simulink model "KeylessStart_harness"  (Simulink 7.7)
settings: Solver=FixedStepDiscrete  SolverMode=SingleTasking  StartTime=0.0  StopTime=100  FixedStep=.01  RelTol=1e-3
PostLoadFcn:
  | cd '..';
  | PostLoadFcn;
  | cd 'harness';
undefined symbols (not defined in the file): sigbuilder_block, srate
libraries: simulink x3
settings Model: Creator=smindema  LastModifiedBy=aliebel  CovMetricSettings=dcmw  CovHTMLOptions=-aTS=1 -bRG=1 -bTC=1 -hTR=0 -nFC=0 -scm=1 -bcm=1 -xEv=0  covSaveCumulativeToWorkspaceVar=off  CovSaveSingleToWorkspaceVar=off
settings MATStruct: SampleTime=0.01  Offset=0  Priority=[1.0]
settings DataIOCC: LimitDataPoints=off  SaveOutput=off  SaveTime=off
settings OptimizationCC: BlockReduction=off  InlineParams=on  ExpressionFolding=off  StateBitsets=on  DataBitsets=on  UseTempVars=on  InitFltsAndDblsToZero=on  NoFixptDivByZeroProtection=on  EfficientFloat2IntCast=on  OptimizeModelRefInitCode=on
settings DebuggingCC: SaveWithParameterizedLinksMsg=none  MultiTaskDSMMsg=warning  MultiTaskCondExecSysMsg=none  IntegerOverflowMsg=none  ModelReferenceCSMismatchMessage=warning
settings HardwareCC: ProdBitPerInt=16  ProdBitPerPointer=16  ProdIntDivRoundTo=Floor  ProdEndianess=BigEndian  ProdWordSize=16  ProdHWDeviceType=Motorola HC12
settings ModelReferenceCC: ModelReferenceNumInstancesAllowed=Single
settings RTWCC: SystemTargetFile=ert.tlc  GenCodeOnly=on  TemplateMakefile=ert_default_tmf  Description=Real-Time Workshop Embedded Coder (no auto configuration)  GenerateReport=on  RetainRTWFile=on  ProcessScript=ert_make_rtw_hook  IncludeHyperlinkInReport=on  LaunchReport=on  IncludeERTFirstTime=on
settings RTWCC: CustomHeaderCode=|
  | #include "cpp_req_defines.h"
  | #include "hw_fin.h"
  | #include "cdata.h"
settings CodeAppCC: IgnoreCustomStorageClasses=off  DefineNamingRule=UpperCase
settings ERTTargetCC: TargetFcnLib=ansi_tfl_tmw.mat  FunctionExecutionProfile=off  MultiwordLength=2048  GenerateSampleERTMain=on  IncludeMdlTerminateFcn=off  SupportAbsoluteTime=off  SupportNonFinite=off  SupportComplex=off  PurelyIntegerCode=on  ERTCustomFileTemplate=gen_rtw_req_defines_h.tlc  GlobalDataDefinition=InSeparateSourceFile  GlobalDataReference=InSeparateHeaderFile  ConvertIfToSwitch=off

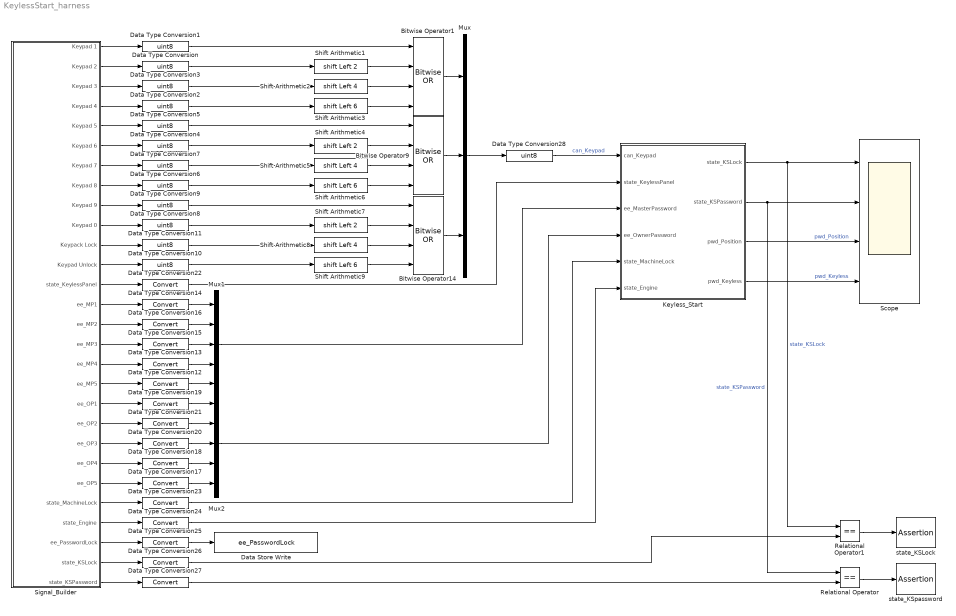
== system KeylessStart_harness ==
  Bitwise Operator1 : simulink/Logic and Bit Operations/Bitwise Operator  logicop=OR  UseBitMask=off  NumInputPorts=4  BitMask=bin2dec('11011001')  BitMaskRealWorld=Stored Integer
  Bitwise Operator14 : simulink/Logic and Bit Operations/Bitwise Operator  logicop=OR  UseBitMask=off  NumInputPorts=4  BitMask=bin2dec('11011001')  BitMaskRealWorld=Stored Integer
  Bitwise Operator9 : simulink/Logic and Bit Operations/Bitwise Operator  logicop=OR  UseBitMask=off  NumInputPorts=4  BitMask=bin2dec('11011001')  BitMaskRealWorld=Stored Integer
  Data Store Write : DataStoreWrite  DataStoreName=ee_PasswordLock
  Data Type Conversion{,1..11,28} (13 alike) : DataTypeConversion  OutDataTypeStr=uint8
  Data Type Conversion{12..27} (16 alike) : DataTypeConversion
  Keyless_Start : Subsystem  TreatAsAtomicUnit=on  SystemSampleTime=srate  RTWFileName=mod_System
      settings: RTWSystemCode=Function  RTWFileNameOpts=User specified
  Mux : Mux  Inputs=3
  Mux1 : Mux  Inputs=5
  Mux2 : Mux  Inputs=5
  Relational Operator : RelationalOperator  Operator===  OutDataTypeStr=boolean
  Relational Operator1 : RelationalOperator  Operator===  OutDataTypeStr=boolean
  Scope : Scope  NumInputPorts=4
      settings: TimeRange=100  YMin=0~0~0~0  YMax=6~10~6~60  DataFormat=Array
  Shift Arithmetic1 : ArithShift  BitShiftNumber=2  BitShiftDirection=Left
  Shift Arithmetic2 : ArithShift  BitShiftNumber=4  BitShiftDirection=Left
  Shift Arithmetic3 : ArithShift  BitShiftNumber=6  BitShiftDirection=Left
  Shift Arithmetic4 : ArithShift  BitShiftNumber=2  BitShiftDirection=Left
  Shift Arithmetic5 : ArithShift  BitShiftNumber=4  BitShiftDirection=Left
  Shift Arithmetic6 : ArithShift  BitShiftNumber=6  BitShiftDirection=Left
  Shift Arithmetic7 : ArithShift  BitShiftNumber=2  BitShiftDirection=Left
  Shift Arithmetic8 : ArithShift  BitShiftNumber=4  BitShiftDirection=Left
  Shift Arithmetic9 : ArithShift  BitShiftNumber=6  BitShiftDirection=Left
  Signal_Builder : Subsystem  Tag=STV Subsys  LoadFcn=sigbuilder_block('load');  StartFcn=sigbuilder_block('start');  StopFcn=sigbuilder_block('stop');  ClipboardFcn=sigbuilder_block('clipboard');  mask(Sigbuilder block){}
      mask help: Sigbuilder GUI
      mask init:
      | if ~strcmp(get_param(bdroot(gcbh),'SimulationStatus'),'stopped') tuvar = sigbuilder_block('maskInit'); end
      settings: CopyFcn=sigbuilder_block('copy');  DeleteFcn=sigbuilder_block('delete');  ModelCloseFcn=sigbuilder_block('modelClose');  PreSaveFcn=sigbuilder_block('preSave');  NameChangeFcn=sigbuilder_block('namechange');  OpenFcn=sigbuilder_block('open',[126.75 84.75 1007.25 697.5 ]);  CloseFcn=sigbuilder_block('close');
      mask Display: plot(0,0,100,100,[10,10,40,40,10],[80,20,20,80,80],[40,10],[50,50], [40,27,10],[65,72,56],[40,25,25,10],[28,28,43,43]);
  state_KSLock : Assertion  Enabled=off
  state_KSpassword : Assertion  Enabled=off
  wires:
  Signal_Builder/2(Keypad 2) -> Data Type Conversion/1
  Relational Operator/1 -> state_KSpassword/1
  Signal_Builder/1(Keypad 1) -> Data Type Conversion1/1
  Bitwise Operator1/1 -> Mux/1
  Shift Arithmetic1/1 -> Bitwise Operator1/2
  Shift Arithmetic2/1 -> Bitwise Operator1/3
  Shift Arithmetic3/1 -> Bitwise Operator1/4
  Shift Arithmetic4/1 -> Bitwise Operator9/2
  Shift Arithmetic5/1 -> Bitwise Operator9/3
  Shift Arithmetic6/1 -> Bitwise Operator9/4
  Bitwise Operator9/1 -> Mux/2
  Bitwise Operator14/1 -> Mux/3
  Shift Arithmetic7/1 -> Bitwise Operator14/2
  Shift Arithmetic8/1 -> Bitwise Operator14/3
  Shift Arithmetic9/1 -> Bitwise Operator14/4
  Mux/1 -> Data Type Conversion28/1
  Data Type Conversion1/1 -> Bitwise Operator1/1
  Signal_Builder/4(Keypad 4) -> Data Type Conversion2/1
  Signal_Builder/5(Keypad 5) -> Data Type Conversion5/1
  Signal_Builder/6(Keypad 6) -> Data Type Conversion4/1
  Signal_Builder/7(Keypad 7) -> Data Type Conversion7/1
  Signal_Builder/8(Keypad 8) -> Data Type Conversion6/1
  Signal_Builder/9(Keypad 9) -> Data Type Conversion9/1
  Signal_Builder/11(Keypack Lock) -> Data Type Conversion11/1
  Signal_Builder/12(Keypad Unlock) -> Data Type Conversion10/1
  Signal_Builder/13(state_KeylessPanel) -> Data Type Conversion22/1
  Mux1/1 -> Keyless_Start/3(ee_MasterPassword)
  Signal_Builder/14(ee_MP1) -> Data Type Conversion14/1
  Signal_Builder/15(ee_MP2) -> Data Type Conversion16/1
  Signal_Builder/16(ee_MP3) -> Data Type Conversion15/1
  Signal_Builder/17(ee_MP4) -> Data Type Conversion13/1
  Signal_Builder/18(ee_MP5) -> Data Type Conversion12/1
  Data Type Conversion14/1 -> Mux1/1
  Data Type Conversion16/1 -> Mux1/2
  Data Type Conversion15/1 -> Mux1/3
  Data Type Conversion13/1 -> Mux1/4
  Data Type Conversion12/1 -> Mux1/5
  Data Type Conversion19/1 -> Mux2/1
  Data Type Conversion21/1 -> Mux2/2
  Data Type Conversion20/1 -> Mux2/3
  Data Type Conversion18/1 -> Mux2/4
  Data Type Conversion17/1 -> Mux2/5
  Signal_Builder/19(ee_OP1) -> Data Type Conversion19/1
  Signal_Builder/20(ee_OP2) -> Data Type Conversion21/1
  Signal_Builder/21(ee_OP3) -> Data Type Conversion20/1
  Signal_Builder/22(ee_OP4) -> Data Type Conversion18/1
  Signal_Builder/23(ee_OP5) -> Data Type Conversion17/1
  Mux2/1 -> Keyless_Start/4(ee_OwnerPassword)
  Signal_Builder/24(state_MachineLock) -> Data Type Conversion23/1
  Signal_Builder/25(state_Engine) -> Data Type Conversion24/1
  Keyless_Start/1(state_KSLock) -> Scope/1, Relational Operator1/1  "state_KSLock"
  Keyless_Start/2(state_KSPassword) -> Relational Operator/1, Scope/2  "state_KSPassword"
  Keyless_Start/3(pwd_Position) -> Scope/3  "pwd_Position"
  Keyless_Start/4(pwd_Keyless) -> Scope/4  "pwd_Keyless"
  Signal_Builder/26(ee_PasswordLock) -> Data Type Conversion25/1
  Relational Operator1/1 -> state_KSLock/1
  Signal_Builder/27(state_KSLock) -> Data Type Conversion26/1
  Signal_Builder/28(state_KSPassword) -> Data Type Conversion27/1
  Data Type Conversion22/1 -> Keyless_Start/2(state_KeylessPanel)
  Data Type Conversion23/1 -> Keyless_Start/5(state_MachineLock)
  Data Type Conversion24/1 -> Keyless_Start/6(state_Engine)
  Data Type Conversion25/1 -> Data Store Write/1
  Data Type Conversion26/1 -> Relational Operator1/2
  Data Type Conversion27/1 -> Relational Operator/2
  Data Type Conversion28/1 -> Keyless_Start/1(can_Keypad)  "can_Keypad"
  Data Type Conversion/1 -> Shift Arithmetic1/1
  Data Type Conversion3/1 -> Shift Arithmetic2/1
  Data Type Conversion2/1 -> Shift Arithmetic3/1
  Data Type Conversion4/1 -> Shift Arithmetic4/1
  Data Type Conversion7/1 -> Shift Arithmetic5/1
  Data Type Conversion6/1 -> Shift Arithmetic6/1
  Data Type Conversion8/1 -> Shift Arithmetic7/1
  Data Type Conversion11/1 -> Shift Arithmetic8/1
  Data Type Conversion10/1 -> Shift Arithmetic9/1
  Data Type Conversion9/1 -> Bitwise Operator14/1
  Data Type Conversion5/1 -> Bitwise Operator9/1
  Signal_Builder/10(Keypad 0) -> Data Type Conversion8/1
  Signal_Builder/3(Keypad 3) -> Data Type Conversion3/1

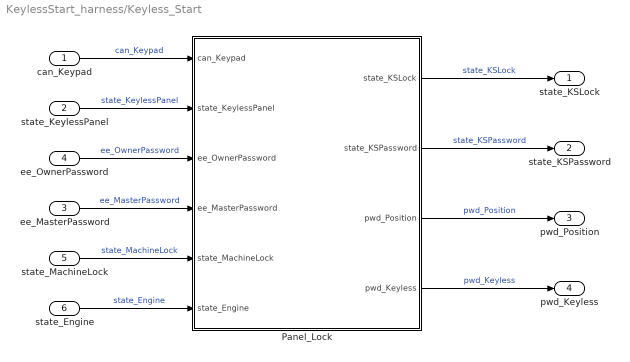
== system KeylessStart_harness/Keyless_Start ==
  can_Keypad : Inport
  state_KeylessPanel : Inport  Port=2
  ee_MasterPassword : Inport  Port=3
  ee_OwnerPassword : Inport  Port=4
  state_MachineLock : Inport  Port=5
  state_Engine : Inport  Port=6
  Panel_Lock : Stateflow chart  TreatAsAtomicUnit=on
  state_KSLock : Outport
  state_KSPassword : Outport  Port=2
  pwd_Position : Outport  Port=3
  pwd_Keyless : Outport  Port=4
  wires:
  can_Keypad/1 -> Panel_Lock/1(can_Keypad)  "can_Keypad"
  state_KeylessPanel/1 -> Panel_Lock/2(state_KeylessPanel)  "state_KeylessPanel"
  Panel_Lock/1(state_KSLock) -> state_KSLock/1  "state_KSLock"
  state_MachineLock/1 -> Panel_Lock/5(state_MachineLock)  "state_MachineLock"
  Panel_Lock/2(state_KSPassword) -> state_KSPassword/1  "state_KSPassword"
  Panel_Lock/3(pwd_Position) -> pwd_Position/1  "pwd_Position"
  Panel_Lock/4(pwd_Keyless) -> pwd_Keyless/1  "pwd_Keyless"
  state_Engine/1 -> Panel_Lock/6(state_Engine)  "state_Engine"
  ee_OwnerPassword/1 -> Panel_Lock/3(ee_OwnerPassword)  "ee_OwnerPassword"
  ee_MasterPassword/1 -> Panel_Lock/4(ee_MasterPassword)  "ee_MasterPassword"

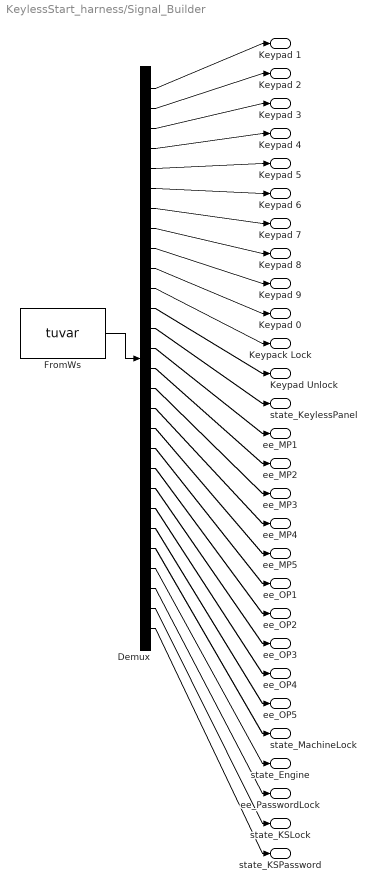
== system KeylessStart_harness/Signal_Builder ==
  Demux : Demux  Tag=STV Demux  Outputs=28
  FromWs : FromWorkspace  Tag=STV FromWs  VariableName=tuvar  SampleTime=0  SigBuilderData=DataTag0  VnvData=DataTag1
      SigBuilderData=|
      | common.afterFinalStr = 'Extrapolate'
      | common.sampleTime = 0
      | dataSet(1).timeRange = [0 100]
      | dataSet(1).name = 'Keypad'
      | dataSet(2).timeRange = [0 100]
      | dataSet(2).name = 'Password'
      | dataSet(3).timeRange = [0 100]
      | dataSet(3).name = 'Password1'
      | dataSet(4).timeRange = [0 100]
      | dataSet(4).name = 'Password2'
      | dataSet(5).timeRange = [0 100]
      | dataSet(5).name = 'Lock'
      | sbobj.Groups(1).Name = 'Keypad'
      | sbobj.Groups(1).Signals(1).Name = 'Keypad 1'
      | sbobj.Groups(1).Signals(1).XData = [0 25 25 26 26 100]
      | sbobj.Groups(1).Signals(1).YData = [0 0 1 1 0 0]
      | sbobj.Groups(1).Signals(2).Name = 'Keypad 2'
      | sbobj.Groups(1).Signals(2).XData = [0 23 23 24 24 100]
      | sbobj.Groups(1).Signals(2).YData = [0 0 1 1 0 0]
      | sbobj.Groups(1).Signals(3).Name = 'Keypad 3'
      | sbobj.Groups(1).Signals(3).XData = [0 21 21 22 22 100]
      | sbobj.Groups(1).Signals(3).YData = [0 0 1 1 0 0]
      | sbobj.Groups(1).Signals(4).Name = 'Keypad 4'
      | sbobj.Groups(1).Signals(4).XData = [0 19 19 20 20 100]
      | sbobj.Groups(1).Signals(4).YData = [0 0 1 1 0 0]
      | sbobj.Groups(1).Signals(5).Name = 'Keypad 5'
      | sbobj.Groups(1).Signals(5).XData = [0 17 17 18 18 100]
      | sbobj.Groups(1).Signals(5).YData = [0 0 1 1 0 0]
      | sbobj.Groups(1).Signals(6).Name = 'Keypad 6'
      | sbobj.Groups(1).Signals(6).XData = [0 13 13 14 14 100]
      | sbobj.Groups(1).Signals(6).YData = [0 0 1 1 0 0]
      | sbobj.Groups(1).Signals(7).Name = 'Keypad 7'
      | sbobj.Groups(1).Signals(7).XData = [0 11 11 12 12 100]
      | sbobj.Groups(1).Signals(7).YData = [0 0 1 1 0 0]
      | sbobj.Groups(1).Signals(8).Name = 'Keypad 8'
      | sbobj.Groups(1).Signals(8).XData = [0 9 9 10 10 100]
      | sbobj.Groups(1).Signals(8).YData = [0 0 1 1 0 0]
      | sbobj.Groups(1).Signals(9).Name = 'Keypad 9'
      | sbobj.Groups(1).Signals(9).XData = [0 7 7 8 8 50 50 51 51 52 52 53 53 54 54 55 55 56 56 57 57 58 58 59 59 61 61 62 62 63 63 64 64 65 65 66 66 67 67 68 68 69 69 70 70 100]
      | sbobj.Groups(1).Signals(9).YData = [0 0 1 1 0 0 1 1 0 0 1 1 0 0 1 1 0 0 1 1 0 0 1 1 0 0 1 1 0 0 1 1 0 0 1 1 0 0 1 1 0 0 1 1 0 0]
      | sbobj.Groups(1).Signals(10).Name = 'Keypad 0'
      | sbobj.Groups(1).Signals(10).XData = [0 5 5 6 6 29 29 30 30 31 31 32 32 33 33 34 34 35 35 36 36 37 37 38 38 100]
      | sbobj.Groups(1).Signals(10).YData = [0 0 1 1 0 0 1 1 0 0 1 1 0 0 1 1 0 0 1 1 0 0 1 1 0 0]
      | sbobj.Groups(1).Signals(11).Name = 'Keypack Lock'
      | sbobj.Groups(1).Signals(11).XData = [0 2 2 4 4 15 15 16 16 27 27 28 28 40 40 41 41 42 42 46 46 100]
      | sbobj.Groups(1).Signals(11).YData = [0 0 1 1 0 0 1 1 0 0 1 1 0 0 1 1 0 0 1 1 0 0]
      | sbobj.Groups(1).Signals(12).Name = 'Keypad Unlock'
      | sbobj.Groups(1).Signals(12).XData = [0 2 2 3 3 40 40 41 41 43 43 46 46 100]
      | sbobj.Groups(1).Signals(12).YData = [0 0 1 1 0 0 1 1 0 0 1 1 0 0]
      | sbobj.Groups(1).Signals(13).Name = 'state_KeylessPanel'
      | sbobj.Groups(1).Signals(13).XData = [0 100]
      | sbobj.Groups(1).Signals(13).YData = [8 8]
      | sbobj.Groups(1).Signals(14).Name = 'ee_MP1'
      | sbobj.Groups(1).Signals(14).XData = [0 100]
      | sbobj.Groups(1).Signals(14).YData = [48 48]
      | sbobj.Groups(1).Signals(15).Name = 'ee_MP2'
      | sbobj.Groups(1).Signals(15).XData = [0 100]
      | sbobj.Groups(1).Signals(15).YData = [48 48]
      | sbobj.Groups(1).Signals(16).Name = 'ee_MP3'
      | sbobj.Groups(1).Signals(16).XData = [0 100]
      | sbobj.Groups(1).Signals(16).YData = [48 48]
      | sbobj.Groups(1).Signals(17).Name = 'ee_MP4'
      | sbobj.Groups(1).Signals(17).XData = [0 100]
      | sbobj.Groups(1).Signals(17).YData = [48 48]
      | sbobj.Groups(1).Signals(18).Name = 'ee_MP5'
      | sbobj.Groups(1).Signals(18).XData = [0 100]
      | sbobj.Groups(1).Signals(18).YData = [48 48]
      | sbobj.Groups(1).Signals(19).Name = 'ee_OP1'
      | sbobj.Groups(1).Signals(19).XData = [0 100]
      | sbobj.Groups(1).Signals(19).YData = [0 0]
      | sbobj.Groups(1).Signals(20).Name = 'ee_OP2'
      | sbobj.Groups(1).Signals(20).XData = [0 100]
      | sbobj.Groups(1).Signals(20).YData = [0 0]
      | sbobj.Groups(1).Signals(21).Name = 'ee_OP3'
      | sbobj.Groups(1).Signals(21).XData = [0 100]
      | sbobj.Groups(1).Signals(21).YData = [0 0]
      | sbobj.Groups(1).Signals(22).Name = 'ee_OP4'
      | sbobj.Groups(1).Signals(22).XData = [0 100]
      | sbobj.Groups(1).Signals(22).YData = [0 0]
      | sbobj.Groups(1).Signals(23).Name = 'ee_OP5'
      | sbobj.Groups(1).Signals(23).XData = [0 100]
      | sbobj.Groups(1).Signals(23).YData = [0 0]
      | sbobj.Groups(1).Signals(24).Name = 'state_MachineLock'
      | sbobj.Groups(1).Signals(24).XData = [0 37.02 37.02 37.03 37.03 100]
      | sbobj.Groups(1).Signals(24).YData = [0 0 1 1 0 0]
      | sbobj.Groups(1).Signals(25).Name = 'state_Engine'
      | sbobj.Groups(1).Signals(25).XData = [0 1 1 100]
      | sbobj.Groups(1).Signals(25).YData = [0 0 1 1]
      | sbobj.Groups(1).Signals(26).Name = 'ee_PasswordLock'
      | sbobj.Groups(1).Signals(26).XData = [0 37.02 37.02 100]
      | sbobj.Groups(1).Signals(26).YData = [0 0 1 1]
      | sbobj.Groups(1).Signals(27).Name = 'state_KSLock'
      | sbobj.Groups(1).Signals(27).XData = [0 0.01 0.02 0.03 0.04 0.05 0.06 0.07 0.08 0.09 0.1 0.11 ... (10001 elements, 1x10001)]
      | sbobj.Groups(1).Signals(27).YData = [0 0 0 0 0 0 0 0 0 0 0 0 ... (10001 elements, 1x10001)]
      | sbobj.Groups(1).Signals(28).Name = 'state_KSPassword'
      | sbobj.Groups(1).Signals(28).XData = [0 0.01 0.02 0.03 0.04 0.05 0.06 0.07 0.08 0.09 0.1 0.11 ... (10001 elements, 1x10001)]
      | sbobj.Groups(1).Signals(28).YData = [0 0 0 0 0 0 0 0 0 0 0 0 ... (10001 elements, 1x10001)]
      | sbobj.Groups(1).TimeRange = [0 100]
      | sbobj.Groups(2).Name = 'Password'
      | sbobj.Groups(2).Signals(1).Name = 'Keypad 1'
      | sbobj.Groups(2).Signals(1).XData = [0 37 37 38 38 49 49 50 50 61 61 62 62 85 85 86 86 100]
      | sbobj.Groups(2).Signals(1).YData = [0 0 1 1 0 0 1 1 0 0 1 1 0 0 1 1 0 0]
      | sbobj.Groups(2).Signals(2).Name = 'Keypad 2'
      | sbobj.Groups(2).Signals(2).XData = [0 51 51 52 52 63 63 64 64 87 87 88 88 100]
      | sbobj.Groups(2).Signals(2).YData = [0 0 1 1 0 0 1 1 0 0 1 1 0 0]
      | sbobj.Groups(2).Signals(3).Name = 'Keypad 3'
      | sbobj.Groups(2).Signals(3).XData = [0 55 55 56 56 65 65 66 66 89 89 90 90 100]
      | sbobj.Groups(2).Signals(3).YData = [0 0 1 1 0 0 1 1 0 0 1 1 0 0]
      | sbobj.Groups(2).Signals(4).Name = 'Keypad 4'
      | sbobj.Groups(2).Signals(4).XData = [0 53 53 54 54 69 69 70 70 91 91 92 92 100]
      | sbobj.Groups(2).Signals(4).YData = [0 0 1 1 0 0 1 1 0 0 1 1 0 0]
      | sbobj.Groups(2).Signals(5).Name = 'Keypad 5'
      | sbobj.Groups(2).Signals(5).XData = [0 57 57 58 58 67 67 68 68 93 94 100]
      | sbobj.Groups(2).Signals(5).YData = [0 0 1 1 0 0 1 1 0 0 0 0]
      | sbobj.Groups(2).Signals(6).Name = 'Keypad 6'
      | sbobj.Groups(2).Signals(6).XData = [0 39 39 40 40 100]
      | sbobj.Groups(2).Signals(6).YData = [0 0 1 1 0 0]
      | sbobj.Groups(2).Signals(7).Name = 'Keypad 7'
      | sbobj.Groups(2).Signals(7).XData = [0 41 41 42 42 100]
      | sbobj.Groups(2).Signals(7).YData = [0 0 1 1 0 0]
      | sbobj.Groups(2).Signals(8).Name = 'Keypad 8'
      | sbobj.Groups(2).Signals(8).XData = [0 43 43 44 44 100]
      | sbobj.Groups(2).Signals(8).YData = [0 0 1 1 0 0]
      | sbobj.Groups(2).Signals(9).Name = 'Keypad 9'
      | sbobj.Groups(2).Signals(9).XData = [0 30 30 33 33 45 45 46 46 77 77 78 78 79 79 80 80 81 81 82 82 100]
      | sbobj.Groups(2).Signals(9).YData = [0 0 1 1 0 0 1 1 0 0 1 1 0 0 1 1 0 0 1 1 0 0]
      | sbobj.Groups(2).Signals(10).Name = 'Keypad 0'
      | sbobj.Groups(2).Signals(10).XData = [0 3 3 4 4 22 22 23 23 24 24 25 25 26 26 27 27 28 28 29 29 30 33 73 73 74 74 75 75 76 76 93 93 94 94 100]
      | sbobj.Groups(2).Signals(10).YData = [0 0 1 1 0 0 1 1 0 0 1 1 0 0 1 1 0 0 1 1 0 0 0 0 1 1 0 0 1 1 0 0 1 1 0 0]
      | sbobj.Groups(2).Signals(11).Name = 'Keypack Lock'
      | sbobj.Groups(2).Signals(11).XData = [0 1 1 2 2 20 20 21 21 35 35 36 36 47 47 48 48 59 59 60 60 71 71 72 72 83 83 84 84 100]
      | sbobj.Groups(2).Signals(11).YData = [0 0 1 1 0 0 1 1 0 0 1 1 0 0 1 1 0 0 1 1 0 0 1 1 0 0 1 1 0 0]
      | sbobj.Groups(2).Signals(12).Name = 'Keypad Unlock'
      | sbobj.Groups(2).Signals(12).XData = [0 100]
      | sbobj.Groups(2).Signals(12).YData = [0 0]
      | sbobj.Groups(2).Signals(13).Name = 'state_KeylessPanel'
      | sbobj.Groups(2).Signals(13).XData = [0 100]
      | sbobj.Groups(2).Signals(13).YData = [8 8]
      | sbobj.Groups(2).Signals(14).Name = 'ee_MP1'
      | sbobj.Groups(2).Signals(14).XData = [0 100]
      | sbobj.Groups(2).Signals(14).YData = [48 48]
      | sbobj.Groups(2).Signals(15).Name = 'ee_MP2'
      | sbobj.Groups(2).Signals(15).XData = [0 100]
      | sbobj.Groups(2).Signals(15).YData = [48 48]
      | sbobj.Groups(2).Signals(16).Name = 'ee_MP3'
      | sbobj.Groups(2).Signals(16).XData = [0 100]
      | sbobj.Groups(2).Signals(16).YData = [48 48]
      | sbobj.Groups(2).Signals(17).Name = 'ee_MP4'
      | sbobj.Groups(2).Signals(17).XData = [0 100]
      | sbobj.Groups(2).Signals(17).YData = [48 48]
      | sbobj.Groups(2).Signals(18).Name = 'ee_MP5'
      | sbobj.Groups(2).Signals(18).XData = [0 100]
      | sbobj.Groups(2).Signals(18).YData = [48 48]
      | sbobj.Groups(2).Signals(19).Name = 'ee_OP1'
      | sbobj.Groups(2).Signals(19).XData = [0 100]
      | sbobj.Groups(2).Signals(19).YData = [49 49]
      | sbobj.Groups(2).Signals(20).Name = 'ee_OP2'
      | sbobj.Groups(2).Signals(20).XData = [0 100]
      | sbobj.Groups(2).Signals(20).YData = [50 50]
      | sbobj.Groups(2).Signals(21).Name = 'ee_OP3'
      | sbobj.Groups(2).Signals(21).XData = [0 100]
      | sbobj.Groups(2).Signals(21).YData = [51 51]
      | sbobj.Groups(2).Signals(22).Name = 'ee_OP4'
      | sbobj.Groups(2).Signals(22).XData = [0 100]
      | sbobj.Groups(2).Signals(22).YData = [52 52]
      | sbobj.Groups(2).Signals(23).Name = 'ee_OP5'
      | sbobj.Groups(2).Signals(23).XData = [0 100]
      | sbobj.Groups(2).Signals(23).YData = [53 53]
      | sbobj.Groups(2).Signals(24).Name = 'state_MachineLock'
      | sbobj.Groups(2).Signals(24).XData = [0 100]
      | sbobj.Groups(2).Signals(24).YData = [0 0]
      | sbobj.Groups(2).Signals(25).Name = 'state_Engine'
      | sbobj.Groups(2).Signals(25).XData = [0 1 1 100]
      | sbobj.Groups(2).Signals(25).YData = [0 0 1 1]
      | sbobj.Groups(2).Signals(26).Name = 'ee_PasswordLock'
      | sbobj.Groups(2).Signals(26).XData = [0 100]
      | sbobj.Groups(2).Signals(26).YData = [0 0]
      | sbobj.Groups(2).Signals(27).Name = 'state_KSLock'
      | sbobj.Groups(2).Signals(27).XData = [0 0.01 0.02 0.03 0.04 0.05 0.06 0.07 0.08 0.09 0.1 0.11 ... (10001 elements, 1x10001)]
      | sbobj.Groups(2).Signals(27).YData = [0 0 0 0 0 0 0 0 0 0 0 0 ... (10001 elements, 1x10001)]
      | sbobj.Groups(2).Signals(28).Name = 'state_KSPassword'
      | sbobj.Groups(2).Signals(28).XData = [0 0.01 0.02 0.03 0.04 0.05 0.06 0.07 0.08 0.09 0.1 0.11 ... (10001 elements, 1x10001)]
      | sbobj.Groups(2).Signals(28).YData = [0 0 0 0 0 0 0 0 0 0 0 0 ... (10001 elements, 1x10001)]
      | sbobj.Groups(2).TimeRange = [0 100]
      | sbobj.Groups(3).Name = 'Password1'
      | sbobj.Groups(3).Signals(1).Name = 'Keypad 1'
      | sbobj.Groups(3).Signals(1).XData = [0 15 15 16 16 49 50 61 62 85 86 100]
      | sbobj.Groups(3).Signals(1).YData = [0 0 1 1 0 0 0 0 0 0 0 0]
      | sbobj.Groups(3).Signals(2).Name = 'Keypad 2'
      | sbobj.Groups(3).Signals(2).XData = [0 17 17 18 18 63 64 87 88 100]
      | sbobj.Groups(3).Signals(2).YData = [0 0 1 1 0 0 0 0 0 0]
      | sbobj.Groups(3).Signals(3).Name = 'Keypad 3'
      | sbobj.Groups(3).Signals(3).XData = [0 19 19 20 20 65 66 89 90 100]
      | sbobj.Groups(3).Signals(3).YData = [0 0 1 1 0 0 0 0 0 0]
      | sbobj.Groups(3).Signals(4).Name = 'Keypad 4'
      | sbobj.Groups(3).Signals(4).XData = [0 21 21 22 22 69 70 91 92 100]
      | sbobj.Groups(3).Signals(4).YData = [0 0 1 1 0 0 0 0 0 0]
      | sbobj.Groups(3).Signals(5).Name = 'Keypad 5'
      | sbobj.Groups(3).Signals(5).XData = [0 23 23 24 24 67 68 93 94 100]
      | sbobj.Groups(3).Signals(5).YData = [0 0 1 1 0 0 0 0 0 0]
      | sbobj.Groups(3).Signals(6).Name = 'Keypad 6'
      | sbobj.Groups(3).Signals(6).XData = [0 39 40 100]
      | sbobj.Groups(3).Signals(6).YData = [0 0 0 0]
      | sbobj.Groups(3).Signals(7).Name = 'Keypad 7'
      | sbobj.Groups(3).Signals(7).XData = [0 41 42 100]
      | sbobj.Groups(3).Signals(7).YData = [0 0 0 0]
      | sbobj.Groups(3).Signals(8).Name = 'Keypad 8'
      | sbobj.Groups(3).Signals(8).XData = [0 43 44 100]
      | sbobj.Groups(3).Signals(8).YData = [0 0 0 0]
      | sbobj.Groups(3).Signals(9).Name = 'Keypad 9'
      | sbobj.Groups(3).Signals(9).XData = [0 9 9 10 10 11 11 12 12 63 63 64 64 79 80 97 97 98 98 100]
      | sbobj.Groups(3).Signals(9).YData = [0 0 1 1 0 0 1 1 0 0 1 1 0 0 0 0 1 1 0 0]
      | sbobj.Groups(3).Signals(10).Name = 'Keypad 0'
      | sbobj.Groups(3).Signals(10).XData = [0 3 3 4 4 5 5 6 6 7 7 8 8 47 47 48 48 49 49 50 50 51 51 52 52 53 53 54 54 55 55 56 56 61 61 62 62 65 65 66 66 67 67 68 68 69 69 70 70 75 76 77 78 81 82 83 84 89 89 90 90 91 91 92 92 93 93 94 94 95 95 96 96 100]
      | sbobj.Groups(3).Signals(10).YData = [0 0 1 1 0 0 1 1 0 0 1 1 0 0 1 1 0 0 1 1 0 0 1 1 0 0 1 1 0 0 1 1 0 0 1 1 0 0 1 1 0 0 1 1 0 0 1 1 0 0 0 0 0 0 0 0 0 0 1 1 0 0 1 1 0 0 1 1 0 0 1 1 0 0]
      | sbobj.Groups(3).Signals(11).Name = 'Keypack Lock'
      | sbobj.Groups(3).Signals(11).XData = [0 1 1 2 2 13 13 14 14 25 25 28 28 43 43 46 46 57 57 60 60 71 74 85 85 88 88 93 94 100]
      | sbobj.Groups(3).Signals(11).YData = [0 0 1 1 0 0 1 1 0 0 1 1 0 0 1 1 0 0 1 1 0 0 0 0 1 1 0 0 0 0]
      | sbobj.Groups(3).Signals(12).Name = 'Keypad Unlock'
      | sbobj.Groups(3).Signals(12).XData = [0 25 25 28 28 43 43 46 46 57 57 60 60 71 74 85 85 88 88 100]
      | sbobj.Groups(3).Signals(12).YData = [0 0 1 1 0 0 1 1 0 0 1 1 0 0 0 0 1 1 0 0]
      | sbobj.Groups(3).Signals(13).Name = 'state_KeylessPanel'
      | sbobj.Groups(3).Signals(13).XData = [0 100]
      | sbobj.Groups(3).Signals(13).YData = [8 8]
      | sbobj.Groups(3).Signals(14).Name = 'ee_MP1'
      | sbobj.Groups(3).Signals(14).XData = [0 100]
      | sbobj.Groups(3).Signals(14).YData = [48 48]
      | sbobj.Groups(3).Signals(15).Name = 'ee_MP2'
      | sbobj.Groups(3).Signals(15).XData = [0 100]
      | sbobj.Groups(3).Signals(15).YData = [48 48]
      | sbobj.Groups(3).Signals(16).Name = 'ee_MP3'
      | sbobj.Groups(3).Signals(16).XData = [0 100]
      | sbobj.Groups(3).Signals(16).YData = [48 48]
      | sbobj.Groups(3).Signals(17).Name = 'ee_MP4'
      | sbobj.Groups(3).Signals(17).XData = [0 100]
      | sbobj.Groups(3).Signals(17).YData = [48 48]
      | sbobj.Groups(3).Signals(18).Name = 'ee_MP5'
      | sbobj.Groups(3).Signals(18).XData = [0 100]
      | sbobj.Groups(3).Signals(18).YData = [48 48]
      | sbobj.Groups(3).Signals(19).Name = 'ee_OP1'
      | sbobj.Groups(3).Signals(19).XData = [0 100]
      | sbobj.Groups(3).Signals(19).YData = [49 49]
      | sbobj.Groups(3).Signals(20).Name = 'ee_OP2'
      | sbobj.Groups(3).Signals(20).XData = [0 100]
      | sbobj.Groups(3).Signals(20).YData = [50 50]
      | sbobj.Groups(3).Signals(21).Name = 'ee_OP3'
      | sbobj.Groups(3).Signals(21).XData = [0 100]
      | sbobj.Groups(3).Signals(21).YData = [51 51]
      | sbobj.Groups(3).Signals(22).Name = 'ee_OP4'
      | sbobj.Groups(3).Signals(22).XData = [0 100]
      | sbobj.Groups(3).Signals(22).YData = [52 52]
      | sbobj.Groups(3).Signals(23).Name = 'ee_OP5'
      | sbobj.Groups(3).Signals(23).XData = [0 100]
      | sbobj.Groups(3).Signals(23).YData = [53 53]
      | sbobj.Groups(3).Signals(24).Name = 'state_MachineLock'
      | sbobj.Groups(3).Signals(24).XData = [0 23.01 23.01 23.02 24.19 24.19 100]
      | sbobj.Groups(3).Signals(24).YData = [0 0 1 1 1 0 0]
      | sbobj.Groups(3).Signals(25).Name = 'state_Engine'
      | sbobj.Groups(3).Signals(25).XData = [0 1 1 100]
      | sbobj.Groups(3).Signals(25).YData = [0 0 1 1]
      | sbobj.Groups(3).Signals(26).Name = 'ee_PasswordLock'
      | sbobj.Groups(3).Signals(26).XData = [0 23.02 23.02 29.1 100]
      | sbobj.Groups(3).Signals(26).YData = [0 0 1 1 1]
      | sbobj.Groups(3).Signals(27).Name = 'state_KSLock'
      | sbobj.Groups(3).Signals(27).XData = [0 0.01 0.02 0.03 0.04 0.05 0.06 0.07 0.08 0.09 0.1 0.11 ... (10001 elements, 1x10001)]
      | sbobj.Groups(3).Signals(27).YData = [0 0 0 0 0 0 0 0 0 0 0 0 ... (10001 elements, 1x10001)]
      | sbobj.Groups(3).Signals(28).Name = 'state_KSPassword'
      | sbobj.Groups(3).Signals(28).XData = [0 0.01 0.02 0.03 0.04 0.05 0.06 0.07 0.08 0.09 0.1 0.11 ... (10001 elements, 1x10001)]
      | sbobj.Groups(3).Signals(28).YData = [0 0 0 0 0 0 0 0 0 0 0 0 ... (10001 elements, 1x10001)]
      | sbobj.Groups(3).TimeRange = [0 100]
      | sbobj.Groups(4).Name = 'Password2'
      | sbobj.Groups(4).Signals(1).Name = 'Keypad 1'
      | sbobj.Groups(4).Signals(1).XData = [0 47 49 50 61 62 85 86 100]
      | sbobj.Groups(4).Signals(1).YData = [0 0 0 0 0 0 0 0 0]
      | sbobj.Groups(4).Signals(2).Name = 'Keypad 2'
      | sbobj.Groups(4).Signals(2).XData = [0 43 45 63 64 87 88 100]
      | sbobj.Groups(4).Signals(2).YData = [0 0 0 0 0 0 0 0]
      | sbobj.Groups(4).Signals(3).Name = 'Keypad 3'
      | sbobj.Groups(4).Signals(3).XData = [0 39 41 65 66 89 90 100]
      | sbobj.Groups(4).Signals(3).YData = [0 0 0 0 0 0 0 0]
      | sbobj.Groups(4).Signals(4).Name = 'Keypad 4'
      | sbobj.Groups(4).Signals(4).XData = [0 36 37 69 70 91 92 100]
      | sbobj.Groups(4).Signals(4).YData = [0 0 0 0 0 0 0 0]
      | sbobj.Groups(4).Signals(5).Name = 'Keypad 5'
      | sbobj.Groups(4).Signals(5).XData = [0 37 38 67 68 93 94 100]
      | sbobj.Groups(4).Signals(5).YData = [0 0 0 0 0 0 0 0]
      | sbobj.Groups(4).Signals(6).Name = 'Keypad 6'
      | sbobj.Groups(4).Signals(6).XData = [0 39 40 100]
      | sbobj.Groups(4).Signals(6).YData = [0 0 0 0]
      | sbobj.Groups(4).Signals(7).Name = 'Keypad 7'
      | sbobj.Groups(4).Signals(7).XData = [0 41 42 100]
      | sbobj.Groups(4).Signals(7).YData = [0 0 0 0]
      | sbobj.Groups(4).Signals(8).Name = 'Keypad 8'
      | sbobj.Groups(4).Signals(8).XData = [0 43 44 100]
      | sbobj.Groups(4).Signals(8).YData = [0 0 0 0]
      | sbobj.Groups(4).Signals(9).Name = 'Keypad 9'
      | sbobj.Groups(4).Signals(9).XData = [0 9 9 10 10 35 35 36 36 46 46 47 47 79 80 97 98 100]
      | sbobj.Groups(4).Signals(9).YData = [0 0 1 1 0 0 1 1 0 0 1 1 0 0 0 0 0 0]
      | sbobj.Groups(4).Signals(10).Name = 'Keypad 0'
      | sbobj.Groups(4).Signals(10).XData = [0 5 5 6 6 7 7 8 8 11 11 12 12 13 13 14 14 15 15 16 16 17 17 18 18 19 19 20 20 21 21 22 22 23 23 24 24 29 29 30 30 31 31 32 32 33 33 34 34 37 37 38 38 40 40 41 41 42 42 43 43 44 44 45 45 48 48 49 49 91 92 93 94 95 96 100]
      | sbobj.Groups(4).Signals(10).YData = [0 0 1 1 0 0 1 1 0 0 1 1 0 0 1 1 0 0 1 1 0 0 1 1 0 0 1 1 0 0 1 1 0 0 1 1 0 0 1 1 0 0 1 1 0 0 1 1 0 0 1 1 0 0 1 1 0 0 1 1 0 0 1 1 0 0 1 1 0 0 0 0 0 0 0 0]
      | sbobj.Groups(4).Signals(11).Name = 'Keypack Lock'
      | sbobj.Groups(4).Signals(11).XData = [0 1 1 4 4 13 14 25 25 28 28 53 56 71 74 85 88 93 94 100]
      | sbobj.Groups(4).Signals(11).YData = [0 0 1 1 0 0 0 0 1 1 0 0 0 0 0 0 0 0 0 0]
      | sbobj.Groups(4).Signals(12).Name = 'Keypad Unlock'
      | sbobj.Groups(4).Signals(12).XData = [0 1 1 4 4 25 25 28 28 71 74 85 88 100]
      | sbobj.Groups(4).Signals(12).YData = [0 0 1 1 0 0 1 1 0 0 0 0 0 0]
      | sbobj.Groups(4).Signals(13).Name = 'state_KeylessPanel'
      | sbobj.Groups(4).Signals(13).XData = [0 100]
      | sbobj.Groups(4).Signals(13).YData = [8 8]
      | sbobj.Groups(4).Signals(14).Name = 'ee_MP1'
      | sbobj.Groups(4).Signals(14).XData = [0 100]
      | sbobj.Groups(4).Signals(14).YData = [48 48]
      | sbobj.Groups(4).Signals(15).Name = 'ee_MP2'
      | sbobj.Groups(4).Signals(15).XData = [0 100]
      | sbobj.Groups(4).Signals(15).YData = [48 48]
      | sbobj.Groups(4).Signals(16).Name = 'ee_MP3'
      | sbobj.Groups(4).Signals(16).XData = [0 100]
      | sbobj.Groups(4).Signals(16).YData = [48 48]
      | sbobj.Groups(4).Signals(17).Name = 'ee_MP4'
      | sbobj.Groups(4).Signals(17).XData = [0 100]
      | sbobj.Groups(4).Signals(17).YData = [48 48]
      | sbobj.Groups(4).Signals(18).Name = 'ee_MP5'
      | sbobj.Groups(4).Signals(18).XData = [0 100]
      | sbobj.Groups(4).Signals(18).YData = [48 48]
      | sbobj.Groups(4).Signals(19).Name = 'ee_OP1'
      | sbobj.Groups(4).Signals(19).XData = [0 48.02 48.02 100]
      | sbobj.Groups(4).Signals(19).YData = [49 49 48 48]
      | sbobj.Groups(4).Signals(20).Name = 'ee_OP2'
      | sbobj.Groups(4).Signals(20).XData = [0 48.02 48.02 100]
      | sbobj.Groups(4).Signals(20).YData = [50 50 48 48]
      | sbobj.Groups(4).Signals(21).Name = 'ee_OP3'
      | sbobj.Groups(4).Signals(21).XData = [0 48.02 48.02 100]
      | sbobj.Groups(4).Signals(21).YData = [51 51 48 48]
      | sbobj.Groups(4).Signals(22).Name = 'ee_OP4'
      | sbobj.Groups(4).Signals(22).XData = [0 48.02 48.02 100]
      | sbobj.Groups(4).Signals(22).YData = [52 52 57 57]
      | sbobj.Groups(4).Signals(23).Name = 'ee_OP5'
      | sbobj.Groups(4).Signals(23).XData = [0 48.02 48.02 100]
      | sbobj.Groups(4).Signals(23).YData = [53 53 48 48]
      | sbobj.Groups(4).Signals(24).Name = 'state_MachineLock'
      | sbobj.Groups(4).Signals(24).XData = [0 23.01 24.19 100]
      | sbobj.Groups(4).Signals(24).YData = [0 0 0 0]
      | sbobj.Groups(4).Signals(25).Name = 'state_Engine'
      | sbobj.Groups(4).Signals(25).XData = [0 1 1 100]
      | sbobj.Groups(4).Signals(25).YData = [0 0 1 1]
      | sbobj.Groups(4).Signals(26).Name = 'ee_PasswordLock'
      | sbobj.Groups(4).Signals(26).XData = [0 100]
      | sbobj.Groups(4).Signals(26).YData = [0 0]
      | sbobj.Groups(4).Signals(27).Name = 'state_KSLock'
      | sbobj.Groups(4).Signals(27).XData = [0 0.01 0.02 0.03 0.04 0.05 0.06 0.07 0.08 0.09 0.1 0.11 ... (10001 elements, 1x10001)]
      | sbobj.Groups(4).Signals(27).YData = [0 0 0 0 0 0 0 0 0 0 0 0 ... (10001 elements, 1x10001)]
      | sbobj.Groups(4).Signals(28).Name = 'state_KSPassword'
      | sbobj.Groups(4).Signals(28).XData = [0 0.01 0.02 0.03 0.04 0.05 0.06 0.07 0.08 0.09 0.1 0.11 ... (10001 elements, 1x10001)]
      | sbobj.Groups(4).Signals(28).YData = [0 0 0 0 0 0 0 0 0 0 0 0 ... (10001 elements, 1x10001)]
      | sbobj.Groups(4).TimeRange = [0 100]
      | sbobj.Groups(5).Name = 'Lock'
      | sbobj.Groups(5).Signals(1).Name = 'Keypad 1'
      | sbobj.Groups(5).Signals(1).XData = [0 26 26 27 27 49 50 61 62 85 86 100]
      | sbobj.Groups(5).Signals(1).YData = [0 0 1 1 0 0 0 0 0 0 0 0]
      | sbobj.Groups(5).Signals(2).Name = 'Keypad 2'
      | sbobj.Groups(5).Signals(2).XData = [0 28 28 29 29 63 64 87 88 100]
      | sbobj.Groups(5).Signals(2).YData = [0 0 1 1 0 0 0 0 0 0]
      | sbobj.Groups(5).Signals(3).Name = 'Keypad 3'
      | sbobj.Groups(5).Signals(3).XData = [0 30 30 31 31 65 66 89 90 100]
      | sbobj.Groups(5).Signals(3).YData = [0 0 1 1 0 0 0 0 0 0]
      | sbobj.Groups(5).Signals(4).Name = 'Keypad 4'
      | sbobj.Groups(5).Signals(4).XData = [0 32 32 33 33 69 70 91 92 100]
      | sbobj.Groups(5).Signals(4).YData = [0 0 1 1 0 0 0 0 0 0]
      | sbobj.Groups(5).Signals(5).Name = 'Keypad 5'
      | sbobj.Groups(5).Signals(5).XData = [0 34 34 35 35 67 68 93 94 100]
      | sbobj.Groups(5).Signals(5).YData = [0 0 1 1 0 0 0 0 0 0]
      | sbobj.Groups(5).Signals(6).Name = 'Keypad 6'
      | sbobj.Groups(5).Signals(6).XData = [0 39 40 100]
      | sbobj.Groups(5).Signals(6).YData = [0 0 0 0]
      | sbobj.Groups(5).Signals(7).Name = 'Keypad 7'
      | sbobj.Groups(5).Signals(7).XData = [0 41 42 100]
      | sbobj.Groups(5).Signals(7).YData = [0 0 0 0]
      | sbobj.Groups(5).Signals(8).Name = 'Keypad 8'
      | sbobj.Groups(5).Signals(8).XData = [0 43 44 100]
      | sbobj.Groups(5).Signals(8).YData = [0 0 0 0]
      | sbobj.Groups(5).Signals(9).Name = 'Keypad 9'
      | sbobj.Groups(5).Signals(9).XData = [0 20 23 27 29 63 63 64 64 79 80 97 97 98 98 100]
      | sbobj.Groups(5).Signals(9).YData = [0 0 0 0 0 0 1 1 0 0 0 0 1 1 0 0]
      | sbobj.Groups(5).Signals(10).Name = 'Keypad 0'
      | sbobj.Groups(5).Signals(10).XData = [0 23 25 28 30 32 35 47 48 49 50 51 52 53 54 55 56 61 61 62 62 65 65 66 66 67 67 68 68 69 69 70 70 75 76 77 78 81 82 83 84 89 89 90 90 91 91 92 92 93 93 94 94 95 95 96 96 100]
      | sbobj.Groups(5).Signals(10).YData = [0 0 0 0 0 0 0 0 0 0 0 0 0 0 0 0 0 0 1 1 0 0 1 1 0 0 1 1 0 0 1 1 0 0 0 0 0 0 0 0 0 0 1 1 0 0 1 1 0 0 1 1 0 0 1 1 0 0]
      | sbobj.Groups(5).Signals(11).Name = 'Keypack Lock'
      | sbobj.Groups(5).Signals(11).XData = [0 1 1 2 2 5 5 6 6 8 8 9 9 11 11 12 12 14 14 15 15 17 17 18 18 20 20 21 21 24 24 25 25 40 40 41 41 93 94 100]
      | sbobj.Groups(5).Signals(11).YData = [0 0 1 1 0 0 1 1 0 0 1 1 0 0 1 1 0 0 1 1 0 0 1 1 0 0 1 1 0 0 1 1 0 0 1 1 0 0 0 0]
      | sbobj.Groups(5).Signals(12).Name = 'Keypad Unlock'
      | sbobj.Groups(5).Signals(12).XData = [0 1 1 2 2 5 5 6 6 8 8 9 9 11 11 13 13 40 40 41 41 43 43 44 44 46 46 47 47 49 49 50 50 60 60 61 61 100]
      | sbobj.Groups(5).Signals(12).YData = [0 0 1 1 0 0 1 1 0 0 1 1 0 0 1 1 0 0 1 1 0 0 1 1 0 0 1 1 0 0 1 1 0 0 1 1 0 0]
      | sbobj.Groups(5).Signals(13).Name = 'state_KeylessPanel'
      | sbobj.Groups(5).Signals(13).XData = [0 4.3 4.3 6.5 6.5 8.4 8.4 9.8 9.8 13 13 15 15 42 42 44 44 100]
      | sbobj.Groups(5).Signals(13).YData = [8 8 4 4 8 8 4 4 8 8 3.8 3.8 8 8 4 4 8 8]
      | sbobj.Groups(5).Signals(14).Name = 'ee_MP1'
      | sbobj.Groups(5).Signals(14).XData = [0 100]
      | sbobj.Groups(5).Signals(14).YData = [48 48]
      | sbobj.Groups(5).Signals(15).Name = 'ee_MP2'
      | sbobj.Groups(5).Signals(15).XData = [0 100]
      | sbobj.Groups(5).Signals(15).YData = [48 48]
      | sbobj.Groups(5).Signals(16).Name = 'ee_MP3'
      | sbobj.Groups(5).Signals(16).XData = [0 100]
      | sbobj.Groups(5).Signals(16).YData = [48 48]
      | sbobj.Groups(5).Signals(17).Name = 'ee_MP4'
      | sbobj.Groups(5).Signals(17).XData = [0 100]
      | sbobj.Groups(5).Signals(17).YData = [48 48]
      | sbobj.Groups(5).Signals(18).Name = 'ee_MP5'
      | sbobj.Groups(5).Signals(18).XData = [0 100]
      | sbobj.Groups(5).Signals(18).YData = [48 48]
      | sbobj.Groups(5).Signals(19).Name = 'ee_OP1'
      | sbobj.Groups(5).Signals(19).XData = [0 100]
      | sbobj.Groups(5).Signals(19).YData = [49 49]
      | sbobj.Groups(5).Signals(20).Name = 'ee_OP2'
      | sbobj.Groups(5).Signals(20).XData = [0 100]
      | sbobj.Groups(5).Signals(20).YData = [50 50]
      | sbobj.Groups(5).Signals(21).Name = 'ee_OP3'
      | sbobj.Groups(5).Signals(21).XData = [0 100]
      | sbobj.Groups(5).Signals(21).YData = [51 51]
      | sbobj.Groups(5).Signals(22).Name = 'ee_OP4'
      | sbobj.Groups(5).Signals(22).XData = [0 100]
      | sbobj.Groups(5).Signals(22).YData = [52 52]
      | sbobj.Groups(5).Signals(23).Name = 'ee_OP5'
      | sbobj.Groups(5).Signals(23).XData = [0 100]
      | sbobj.Groups(5).Signals(23).YData = [53 53]
      | sbobj.Groups(5).Signals(24).Name = 'state_MachineLock'
      | sbobj.Groups(5).Signals(24).XData = [0 34 34 37.97 37.97 100]
      | sbobj.Groups(5).Signals(24).YData = [0 0 1 1 0 0]
      | sbobj.Groups(5).Signals(25).Name = 'state_Engine'
      | sbobj.Groups(5).Signals(25).XData = [0 3 3 16 16 18 18 45 45 47 47 100]
      | sbobj.Groups(5).Signals(25).YData = [0 0 1 1 2 2 1 1 2 2 1 1]
      | sbobj.Groups(5).Signals(26).Name = 'ee_PasswordLock'
      | sbobj.Groups(5).Signals(26).XData = [0 20.6 20.6 21.6 21.6 34 34 34.02 34.02 37 37 37.01 37.01 42.4 42.4 50.9 50.9 59.6 59.6 100]
      | sbobj.Groups(5).Signals(26).YData = [0 0 1 1 0 0 1 1 0 0 1 1 0 0 1 1 0 0 1 1]
      | sbobj.Groups(5).Signals(27).Name = 'state_KSLock'
      | sbobj.Groups(5).Signals(27).XData = [0 0.01 0.02 0.03 0.04 0.05 0.06 0.07 0.08 0.09 0.1 0.11 ... (10001 elements, 1x10001)]
      | sbobj.Groups(5).Signals(27).YData = [0 0 0 0 0 0 0 0 0 0 0 0 ... (10001 elements, 1x10001)]
      | sbobj.Groups(5).Signals(28).Name = 'state_KSPassword'
      | sbobj.Groups(5).Signals(28).XData = [0 0.01 0.02 0.03 0.04 0.05 0.06 0.07 0.08 0.09 0.1 0.11 ... (10001 elements, 1x10001)]
      | sbobj.Groups(5).Signals(28).YData = [0 0 0 0 0 0 0 0 0 0 0 0 ... (10001 elements, 1x10001)]
      | sbobj.Groups(5).TimeRange = [0 100]
  Keypad 1 : Outport  Tag=STV Outport
  Keypad 2 : Outport  Tag=STV Outport  Port=2
  Keypad 3 : Outport  Tag=STV Outport  Port=3
  Keypad 4 : Outport  Tag=STV Outport  Port=4
  Keypad 5 : Outport  Tag=STV Outport  Port=5
  Keypad 6 : Outport  Tag=STV Outport  Port=6
  Keypad 7 : Outport  Tag=STV Outport  Port=7
  Keypad 8 : Outport  Tag=STV Outport  Port=8
  Keypad 9 : Outport  Tag=STV Outport  Port=9
  Keypad 0 : Outport  Tag=STV Outport  Port=10
  Keypack Lock : Outport  Tag=STV Outport  Port=11
  Keypad Unlock : Outport  Tag=STV Outport  Port=12
  state_KeylessPanel : Outport  Tag=STV Outport  Port=13
  ee_MP1 : Outport  Tag=STV Outport  Port=14
  ee_MP2 : Outport  Tag=STV Outport  Port=15
  ee_MP3 : Outport  Tag=STV Outport  Port=16
  ee_MP4 : Outport  Tag=STV Outport  Port=17
  ee_MP5 : Outport  Tag=STV Outport  Port=18
  ee_OP1 : Outport  Tag=STV Outport  Port=19
  ee_OP2 : Outport  Tag=STV Outport  Port=20
  ee_OP3 : Outport  Tag=STV Outport  Port=21
  ee_OP4 : Outport  Tag=STV Outport  Port=22
  ee_OP5 : Outport  Tag=STV Outport  Port=23
  state_MachineLock : Outport  Tag=STV Outport  Port=24
  state_Engine : Outport  Tag=STV Outport  Port=25
  ee_PasswordLock : Outport  Tag=STV Outport  Port=26
  state_KSLock : Outport  Tag=STV Outport  Port=27
  state_KSPassword : Outport  Tag=STV Outport  Port=28
  wires:
  FromWs/1 -> Demux/1
  Demux/1 -> Keypad 1/1
  Demux/2 -> Keypad 2/1
  Demux/3 -> Keypad 3/1
  Demux/4 -> Keypad 4/1
  Demux/5 -> Keypad 5/1
  Demux/6 -> Keypad 6/1
  Demux/7 -> Keypad 7/1
  Demux/8 -> Keypad 8/1
  Demux/9 -> Keypad 9/1
  Demux/10 -> Keypad 0/1
  Demux/11 -> Keypack Lock/1
  Demux/12 -> Keypad Unlock/1
  Demux/13 -> state_KeylessPanel/1
  Demux/14 -> ee_MP1/1
  Demux/15 -> ee_MP2/1
  Demux/16 -> ee_MP3/1
  Demux/17 -> ee_MP4/1
  Demux/18 -> ee_MP5/1
  Demux/19 -> ee_OP1/1
  Demux/20 -> ee_OP2/1
  Demux/21 -> ee_OP3/1
  Demux/22 -> ee_OP4/1
  Demux/23 -> ee_OP5/1
  Demux/24 -> state_MachineLock/1
  Demux/25 -> state_Engine/1
  Demux/26 -> ee_PasswordLock/1
  Demux/27 -> state_KSLock/1
  Demux/28 -> state_KSPassword/1

== stateflow chart Keyless_Start/Panel_Lock ==
  state KS_LOCK [parallel]
    settings: executionOrder=3
    state LOCK
      en:state_KSLock = KS_LOCK_MACHINE;
    state UNLOCK
      en:state_KSLock = KS_UNLOCK_MACHINE;
    state NOTHING
      en:state_KSLock = KS_NOTHING;
    state BUTTON_CHANGE_DB
      en:debounceCount = 0;
      du:debounceCount++;
    state CHANGE
      en:state_KSLock = KS_CHANGE;
    state MACHINE_LOCK
      en:state_KSLock = KS_LOCK;
    state MACHINE_UNLOCK
      en:state_KSLock = KS_UNLOCK;
    KS_LOCK.NOTHING -> LOCK [order 4] : [((can_Keypad[2] & KEYPAD_LOCK_MASK) == KEYPAD_LOCK_PRESSED)...
        | && ((can_Keypad[2] & KEYPAD_UNLOCK_MASK) == 0)...
        | && (ee_PasswordLock == UNLOCK)...
        | && (state_KeylessPanel == NORMAL)...
        | && (state_Engine == ENGINE_NOT_RUNNING)]
    (default) -> KS_LOCK.NOTHING
    LOCK -> KS_LOCK.NOTHING [order 2] : [(state_KSPassword == FAIL)]
    LOCK -> MACHINE_LOCK [order 1] : [(ee_PasswordLock == LOCKED)]
    KS_LOCK.NOTHING -> UNLOCK [order 2] : [((can_Keypad[2] & KEYPAD_UNLOCK_MASK) == KEYPAD_UNLOCK_PRESSED)...
        | && ((can_Keypad[2] & KEYPAD_LOCK_MASK) == 0)...
        | && (ee_PasswordLock == LOCKED)...
        | && (state_KeylessPanel == NORMAL)...
        | && (state_Engine == ENGINE_NOT_RUNNING)]
    UNLOCK -> KS_LOCK.NOTHING : [(ee_PasswordLock == UNLOCK)...
        | || (state_KSPassword == FAIL)]
    KS_LOCK.NOTHING -> BUTTON_CHANGE_DB [order 3] : [((can_Keypad[2] & KEYPAD_LOCK_MASK) == KEYPAD_LOCK_PRESSED)...
        | && ((can_Keypad[2] & KEYPAD_UNLOCK_MASK) == KEYPAD_UNLOCK_PRESSED)...
        | && (state_KeylessPanel == NORMAL)...
        | && (state_Engine == ENGINE_NOT_RUNNING)]
    BUTTON_CHANGE_DB -> KS_LOCK.NOTHING [order 1] : [((can_Keypad[2] & KEYPAD_LOCK_MASK) == 0)...
        | || ((can_Keypad[2] & KEYPAD_UNLOCK_MASK) == 0)...
        | || (state_KeylessPanel != NORMAL)]
    BUTTON_CHANGE_DB -> CHANGE [order 2] : [(debounceCount >= 200)]
    CHANGE -> KS_LOCK.NOTHING : [(state_KSPassword == NEW)...
        | || (state_KSPassword == FAIL)]
    KS_LOCK.NOTHING -> MACHINE_LOCK [order 1] : [(state_MachineLock == LOCKED)...
        | && (ee_PasswordLock == ACTIVE)]
    MACHINE_LOCK -> MACHINE_UNLOCK [order 2] : [(state_KSPassword == PASS)]
    MACHINE_UNLOCK -> KS_LOCK.NOTHING : [(state_MachineLock == UNLOCK)...
        | || (ee_PasswordLock == INACTIVE)]
    MACHINE_LOCK -> KS_LOCK.NOTHING [order 1] : [(ee_PasswordLock == INACTIVE)]
  state KEYPAD [parallel]
    settings: executionOrder=1
    state NOT_PRESSED
      en:
      reset_PwdState = 0;
    state PRESSED
      state NONE
      state BUTTON_1
        en:pwd_Keyless[pwd_Position] = ASCII_1;
        en:pwd_Position++;
      state BUTTON_0
        en:pwd_Keyless[pwd_Position] = ASCII_0;
        en:pwd_Position++;
      state BUTTON_2
        en:pwd_Keyless[pwd_Position] = ASCII_2;
        en:pwd_Position++;
      state BUTTON_3
        en:pwd_Keyless[pwd_Position] = ASCII_3;
        en:pwd_Position++;
      state BUTTON_4
        en:pwd_Keyless[pwd_Position] = ASCII_4;
        en:pwd_Position++;
      state BUTTON_5
        en:pwd_Keyless[pwd_Position] = ASCII_5;
        en:pwd_Position++;
      state BUTTON_6
        en:pwd_Keyless[pwd_Position] = ASCII_6;
        en:pwd_Position++;
      state BUTTON_74
        en:pwd_Keyless[pwd_Position] = ASCII_7;
        en:pwd_Position++;
      state BUTTON_8
        en:pwd_Keyless[pwd_Position] = ASCII_8;
        en:pwd_Position++;
      state BUTTON_9
        en:pwd_Keyless[pwd_Position] = ASCII_9;
        en:pwd_Position++;
      (default) -> NONE
      NONE -> BUTTON_1 [order 9] : [((can_Keypad[0] & KEYPAD_MASK_1) == KEYPAD_PRESSED_1)]
      NONE -> BUTTON_0 [order 10] : [((can_Keypad[2] & KEYPAD_MASK_0) == KEYPAD_PRESSED_0)]
      NONE -> BUTTON_2 [order 8] : [((can_Keypad[0] & KEYPAD_MASK_2) == KEYPAD_PRESSED_2)]
      NONE -> BUTTON_3 [order 7] : [((can_Keypad[0] & KEYPAD_MASK_3) == KEYPAD_PRESSED_3)]
      NONE -> BUTTON_4 [order 6] : [((can_Keypad[0] & KEYPAD_MASK_4) == KEYPAD_PRESSED_4)]
      NONE -> BUTTON_5 [order 5] : [((can_Keypad[1] & KEYPAD_MASK_5) == KEYPAD_PRESSED_5)]
      NONE -> BUTTON_6 [order 4] : [((can_Keypad[1] & KEYPAD_MASK_6) == KEYPAD_PRESSED_6)]
      NONE -> BUTTON_74 [order 3] : [((can_Keypad[1] & KEYPAD_MASK_7) == KEYPAD_PRESSED_7)]
      NONE -> BUTTON_8 [order 2] : [((can_Keypad[1] & KEYPAD_MASK_8) == KEYPAD_PRESSED_8)]
      NONE -> BUTTON_9 [order 1] : [((can_Keypad[2] & KEYPAD_MASK_9) == KEYPAD_PRESSED_9)]
    state RESET
      en:
      pwd_Position = 0;
      pwd_Keyless = 0;
      reset_PwdState = 1;
    (default) -> NOT_PRESSED
    NOT_PRESSED -> PRESSED [order 1] : [((can_Keypad[0] != 0) || (can_Keypad[1] != 0) || (can_Keypad[2] != 0))...
        | && ((state_KSPassword == ENTER_PWD) || (state_KSPassword == ENTER_OWNER1) || (state_KSPassword == ENTER_OWNER2))]
    PRESSED -> NOT_PRESSED : [(can_Keypad[0] == 0)...
        | && (can_Keypad[1] == 0)...
        | && (can_Keypad[2] == 0)]
    NOT_PRESSED -> RESET [order 2] : [(state_KSPassword == FAIL)]
    RESET -> NOT_PRESSED : [after(200,tick)...
        | && (state_KSPassword != FAIL)]
        | %can't get coverage on this
        | % KSPassword chart will not allow KSPassword to remain in the fail state after 200 tick
  state KS_PASSWORD [parallel]
    settings: executionOrder=2
    state WAIT_NEW
      en:state_KSPassword = ENTER_OWNER2;
    state WAIT_UNLOCK
    state NOTHING
      en:state_KSPassword = KS_NOTHING;
      en:pwd_Position = 0;
      en:pwd_Keyless = 0;
    state WAIT_UNLOCK_CHART
      en:state_KSPassword = ENTER_PWD;
    state GOOD_UNLOCK
      (default) -> (junction 38)
      (junction 38) -> (junction 41) [order 2] : {
          | state_KSPassword = FAIL;
          | }
      (junction 38) -> (junction 39) [order 1] : [((ee_OwnerPassword[0] == pwd_Keyless[0])...
          |    && (ee_OwnerPassword[1] == pwd_Keyless[1])...
          |    && (ee_OwnerPassword[2] == pwd_Keyless[2])...
          |    && (ee_OwnerPassword[3] == pwd_Keyless[3])...
          |    && (ee_OwnerPassword[4] == pwd_Keyless[4]))...
          | || ((ee_MasterPassword[0] == pwd_Keyless[0])...
          |    && (ee_MasterPassword[1] == pwd_Keyless[1])...
          |    && (ee_MasterPassword[2] == pwd_Keyless[2])...
          |    && (ee_MasterPassword[3] == pwd_Keyless[3])...
          |    && (ee_MasterPassword[4] == pwd_Keyless[4]))]
      (junction 39) -> (junction 40) : {
          | state_KSPassword = PASS;
          | }
      (junction 40) -> (junction 41)
    state FAIL
      en:state_KSPassword = FAIL;
    state GOOD_NEW
      en:state_KSPassword = NEW;
    state WAIT_OWNER
      en:state_KSPassword = ENTER_OWNER1;
    state GOOD_CHANGE
      (default) -> (junction 42)
      (junction 42) -> (junction 43) [order 1] : [(pwd_New[0] == pwd_Keyless[0])...
          |    && (pwd_New[1] == pwd_Keyless[1])...
          |    && (pwd_New[2] == pwd_Keyless[2])...
          |    && (pwd_New[3] == pwd_Keyless[3])...
          |    && (pwd_New[4] == pwd_Keyless[4])]
      (junction 42) -> (junction 44) [order 2] : {
          | state_KSPassword = FAIL;
          | }
      (junction 43) -> (junction 45) : {
          | state_KSPassword = PASS;
          | }
      (junction 45) -> (junction 44)
    state GOOD
      (junction 46) -> (junction 49)
      (junction 48) -> (junction 46) : {
          | state_KSPassword = FAIL;
          | }
      (default) -> (junction 47)
      (junction 47) -> (junction 48) [order 1] : [((pwd_Keyless[0] == ASCII_0)...
          |    && (pwd_Keyless[1] == ASCII_0)...
          |    && (pwd_Keyless[2] == ASCII_0)...
          |    && (pwd_Keyless[3] == ASCII_0)...
          |    && (pwd_Keyless[4] == ASCII_0))]
      (junction 47) -> (junction 49) [order 2] : {
          | pwd_New = pwd_Keyless;
          | pwd_Keyless = 0;
          | pwd_Position = 0;
          | state_KSPassword = PASS;
          | }
    WAIT_UNLOCK_CHART -> WAIT_UNLOCK : [(pwd_Position != 0)]
    (junction 50) -> FAIL
    WAIT_NEW -> (junction 50) [order 1] : [after(CD_KEYPAD_ENTER_TIME,tick)]
    (default) -> KS_PASSWORD.NOTHING
    KS_PASSWORD.NOTHING -> WAIT_UNLOCK_CHART [order 2] : [(state_KSLock != KS_NOTHING)]
    WAIT_UNLOCK -> GOOD_UNLOCK [order 2] : [(pwd_Position == MAX_PWD_CHAR)]
    KS_PASSWORD.NOTHING -> WAIT_OWNER [order 1] : [(state_KSLock == KS_CHANGE)]
    GOOD_CHANGE -> GOOD_NEW [order 1] : [(state_KSPassword == PASS)]
    GOOD_UNLOCK -> FAIL [order 2] : [(state_KSPassword == FAIL)]
    GOOD -> (junction 50) [order 2]
    GOOD_UNLOCK -> (junction 37) [order 1] : [after(50,tick)...
        | &&(state_KSLock == KS_NOTHING)]
        | {
        | pwd_Position = 0;
        | pwd_Keyless = 0;
        | }
    GOOD_NEW -> (junction 37) : [after(50,tick)...
        | && (ee_OwnerPassword[0] == pwd_Keyless[0])...
        | && (ee_OwnerPassword[1] == pwd_Keyless[1])...
        | && (ee_OwnerPassword[2] == pwd_Keyless[2])...
        | && (ee_OwnerPassword[3] == pwd_Keyless[3])...
        | && (ee_OwnerPassword[4] == pwd_Keyless[4])]
    FAIL -> (junction 37) : [after(200,tick)...
        | && (reset_PwdState)]
    (junction 37) -> KS_PASSWORD.NOTHING
    GOOD -> WAIT_NEW [order 1] : [(state_KSPassword == PASS)]
    WAIT_UNLOCK -> FAIL [order 1] : [after(CD_KEYPAD_ENTER_TIME, tick)]
    WAIT_NEW -> GOOD_CHANGE [order 2] : [(pwd_Position == MAX_PWD_CHAR)]
    WAIT_OWNER -> GOOD [order 2] : [(pwd_Position == MAX_PWD_CHAR)]
    GOOD_CHANGE -> (junction 50) [order 2]
    WAIT_OWNER -> (junction 50) [order 1] : [after(CD_KEYPAD_ENTER_TIME, tick)]
  data: can_Keypad input uint8 size=3; state_KeylessPanel input uint8; state_KSLock output uint8; debounceCount local uint16; KEYPAD_LOCK_MASK parameter uint8; KEYPAD_LOCK_PRESSED parameter uint8; KEYPAD_UNLOCK_MASK parameter uint8; KEYPAD_UNLOCK_PRESSED parameter uint8; NORMAL parameter uint8; PASS parameter uint8; FAIL parameter uint8; state_KSPassword output uint8; KS_LOCK parameter uint8; KS_UNLOCK parameter uint8; KS_CHANGE parameter uint8; KS_NOTHING parameter uint8; NEW parameter uint8; LOCKED parameter uint8; UNLOCK parameter uint8; pwd_Position output uint8; pwd_Keyless output uint8 size=5; ASCII_1 parameter uint8; ASCII_2 parameter uint8; ASCII_3 parameter uint8; ASCII_4 parameter uint8; ASCII_5 parameter uint8; ASCII_6 parameter uint8; ASCII_7 parameter uint8; ASCII_8 parameter uint8; ASCII_9 parameter uint8; ASCII_0 parameter uint8; KEYPAD_PRESSED_1 parameter uint8; KEYPAD_MASK_1 parameter uint8; KEYPAD_MASK_2 parameter uint8; KEYPAD_PRESSED_2 parameter uint8; KEYPAD_MASK_3 parameter uint8; KEYPAD_PRESSED_3 parameter uint8; KEYPAD_MASK_4 parameter uint8; KEYPAD_PRESSED_4 parameter uint8; KEYPAD_MASK_5 parameter uint8; KEYPAD_PRESSED_5 parameter uint8; KEYPAD_MASK_6 parameter uint8; KEYPAD_PRESSED_6 parameter uint8; KEYPAD_MASK_7 parameter uint8; KEYPAD_PRESSED_7 parameter uint8; KEYPAD_MASK_8 parameter uint8; KEYPAD_PRESSED_8 parameter uint8; KEYPAD_MASK_9 parameter uint8; KEYPAD_PRESSED_9 parameter uint8; KEYPAD_MASK_0 parameter uint8; KEYPAD_PRESSED_0 parameter uint8; MAX_PWD_CHAR parameter uint8; ee_OwnerPassword input uint8 size=5; ee_MasterPassword input uint8 size=5; reset_PwdState local uint8; state_MachineLock input uint8; KS_LOCK_MACHINE parameter uint8; KS_UNLOCK_MACHINE parameter uint8; ENTER_OWNER1 parameter uint8; ACTIVE parameter uint8; INACTIVE parameter uint8; CD_KEYPAD_ENTER_TIME parameter uint16; pwd_New local uint8 size=5; ENTER_OWNER2 parameter uint8; ENTER_PWD parameter uint8; ENGINE_NOT_RUNNING parameter uint8; state_Engine input uint8; ee_PasswordLock data_store_memory double
